simulink model "es_control_przyklad"  (R2025b)
settings: Solver=FixedStepAuto  StartTime=0.0  StopTime=Inf  FixedStep=0.01  MaxStep=0.001  RelTol=1e-3  EnableMultiTasking=on
libraries: arduinolib x5, simulink x1
settings Model: SimulationMode=external  ExtModeTrigDuration=2  Creator=mirka  LastModifiedBy=USER
settings SolverCC: AutoInsertRateTranBlk=on
settings OptimizationCC: EnhancedBackFolding=on  PassReuseOutputArgsAs=Individual arguments  ZeroExternalMemoryAtStartup=off  ZeroInternalMemoryAtStartup=off  MaxStackSize=64  OptimizeBlockOrder=speed  DifferentSizesBufferReuse=on  OptimizationCustomize=off  EfficientTunableParamExpr=on
settings DebuggingCC: ParameterTunabilityLossMsg=error
settings HardwareCC: ProdBitPerInt=16.0  ProdBitPerPointer=16.0  ProdBitPerSizeT=16.0  ProdBitPerPtrDiffT=16.0  ProdLargestAtomicFloat=None  ProdWordSize=8.0  ProdHWDeviceType=Atmel->AVR  UseEmbeddedCoderFeatures=off  UseSimulinkCoderFeatures=off
settings SFSimCC: MATLABDynamicMemAlloc=off
settings RTWCC: SystemTargetFile=ert.tlc  HardwareBoard=Arduino Uno  TemplateMakefile=ert_default_tmf  Toolchain=Arduino AVR  BuildConfiguration=Faster Runs  Description=Embedded Coder
settings CodeAppCC: ForceParamTrailComments=on  IgnoreCustomStorageClasses=off  OperatorAnnotations=on  SimulinkDataObjDesc=on  SFDataObjDesc=on  InsertBlockDesc=on
settings ERTTargetCC: ExtModeTransport=3.0  ExtModeStaticAlloc=on  ExtModeAutomaticAllocSize=off  ExtModeStaticAllocSize=250.0  ExtModeMexFile=ext_xcp  ExtModeIntrfLevel=Level2 - Open  InlinedParameterPlacement=Hierarchical  SupportContinuousTime=on  SupportNonInlinedSFcns=on  SupportVariableSizeSignals=on

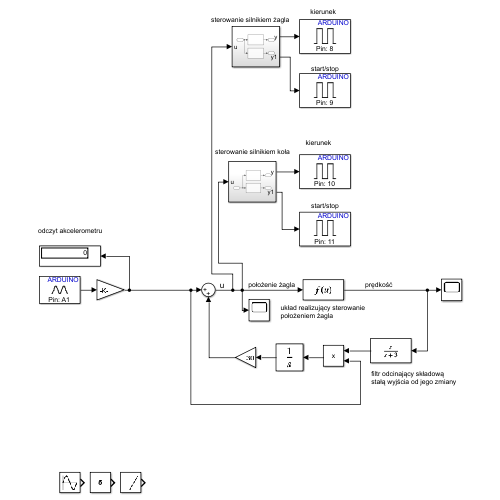
[thumbnail: Simulink's stored preview of the top-level diagram]
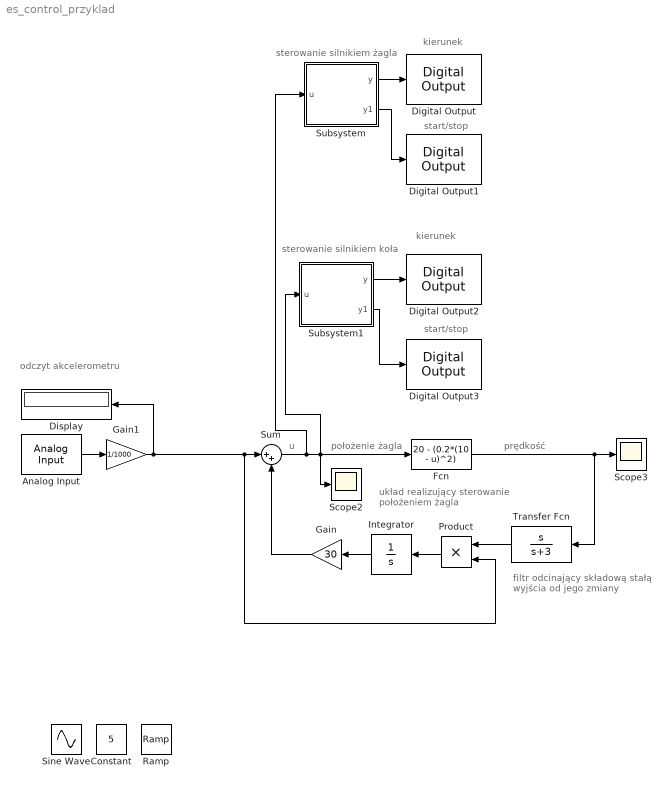
== system es_control_przyklad ==
  note: układ realizujący sterowanie położeniem żagla
  note: prędkość
  note: położenie żagla
  note: filtr odcinający składową stałą wyjścia od jego zmiany
  note: u
  note: odczyt akcelerometru
  note: sterowanie silnikiem żagla
  note: sterowanie silnikiem koła
  note: kierunek
  note: kierunek
  note: start/stop
  note: start/stop
  Analog Input : arduinolib/Analog Input  pinNumber=1  ReadResultsOnly=off  ConversionTriggerSource=Software  ExternalTriggerType=uint32( 0 )  OutputDataType=uint16  EnableConversionCompleteNotify=off  EnableOuputStatus=off  SampleTime=0.01  blockPlatform=arduino
      settings: LibrarySourceBlock=gizmoLibrary/Arduino Utilities/Analog Input
  Constant : Constant  Value=5
  Digital Output : arduinolib/Digital Output  pinNumber=8  Direction=output  blockPlatform=arduino
      settings: LibrarySourceBlock=gizmoLibrary/Arduino Utilities/Digital Output
  Digital Output1 : arduinolib/Digital Output  pinNumber=9  Direction=output  blockPlatform=arduino
      settings: LibrarySourceBlock=gizmoLibrary/Arduino Utilities/Digital Output
  Digital Output2 : arduinolib/Digital Output  pinNumber=10  Direction=output  blockPlatform=arduino
      settings: LibrarySourceBlock=gizmoLibrary/Arduino Utilities/Digital Output
  Digital Output3 : arduinolib/Digital Output  pinNumber=11  Direction=output  blockPlatform=arduino
      settings: LibrarySourceBlock=gizmoLibrary/Arduino Utilities/Digital Output
  Display : Display
  Fcn : Fcn  Expr=20 - (0.2*(10 - u)^2)
  Gain : Gain  Gain=30
  Gain1 : Gain  Gain=1/1000
  Integrator : Integrator
  Product : Product
  Ramp : simulink/Sources/Ramp  slope=2  start=0  InitialOutput=0
  Scope2 : Scope
      settings: ActiveDisplayYMinimum=-109.07087871215685  ActiveDisplayYMaximum=1132.7305074093902  DataLoggingVariableName=ScopeData2
  Scope3 : Scope
      settings: ActiveDisplayYMinimum=-109.07087871215685  ActiveDisplayYMaximum=1132.7305074093902  DataLoggingVariableName=ScopeData3
  Sine Wave : Sin  Amplitude=0.3  Frequency=6  SampleTime=0  VectorParams1D=off
  Subsystem : Subsystem
  Subsystem1 : Subsystem
  Sum : Sum  Inputs=|++
  Transfer Fcn : TransferFcn  Numerator=[1 0]  Denominator=[1 3]
  wires:
  Sum/1 -> Fcn/1, Subsystem1/1(u), Scope2/1, Subsystem/1(u)
  Fcn/1 -> Transfer Fcn/1, Scope3/1
  Transfer Fcn/1 -> Product/1
  Product/1 -> Integrator/1
  Integrator/1 -> Gain/1
  Gain/1 -> Sum/2
  Analog Input/1 -> Gain1/1
  Gain1/1 -> Product/2, Sum/1, Display/1
  Subsystem1/1(y) -> Digital Output2/1
  Subsystem1/2(y1) -> Digital Output3/1
  Subsystem/1(y) -> Digital Output/1
  Subsystem/2(y1) -> Digital Output1/1

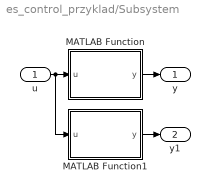
== system es_control_przyklad/Subsystem ==
  u : Inport
  MATLAB Function : MATLAB Function  AncestorBlock=gizmoLibrary/Gizmo Blocks/MATLAB Function  TreatAsAtomicUnit=on
  MATLAB Function1 : MATLAB Function  AncestorBlock=gizmoLibrary/Gizmo Blocks/MATLAB Function  TreatAsAtomicUnit=on
  y : Outport
  y1 : Outport  Port=2
  wires:
  u/1 -> MATLAB Function1/1(u), MATLAB Function/1(u)
  MATLAB Function/1(y) -> y/1
  MATLAB Function1/1(y) -> y1/1

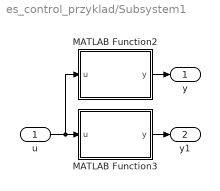
== system es_control_przyklad/Subsystem1 ==
  u : Inport
  MATLAB Function2 : MATLAB Function  AncestorBlock=gizmoLibrary/Gizmo Blocks/MATLAB Function  TreatAsAtomicUnit=on
  MATLAB Function3 : MATLAB Function  AncestorBlock=gizmoLibrary/Gizmo Blocks/MATLAB Function  TreatAsAtomicUnit=on
  y : Outport
  y1 : Outport  Port=2
  wires:
  u/1 -> MATLAB Function2/1(u), MATLAB Function3/1(u)
  MATLAB Function2/1(y) -> y/1
  MATLAB Function3/1(y) -> y1/1

== matlab function es_control_przyklad/Subsystem/MATLAB Function ==
  data: u input; y output
function y = fcn(u)

y = 1;

== matlab function es_control_przyklad/Subsystem1/MATLAB Function2 ==
  data: u input; y output
function y = fcn(u)

y = 0;

== matlab function es_control_przyklad/Subsystem1/MATLAB Function3 ==
  data: u input; y output
function y = fcn(u)

y = 0;

== matlab function es_control_przyklad/Subsystem/MATLAB Function1 ==
  data: u input; y output
function y = fcn(u)

y = 0;
